simulink model "MARCH_v1_4"  (R2016a)
settings: Solver=FixedStepDiscrete  StartTime=0.0  StopTime=inf  FixedStep=0.001  RelTol=1e-3
InitFcn:
  | % Change dir to model location
  | cd(fileparts(which(bdroot)));
  | 
  | init_model
StartFcn:
  | cd(fileparts(which(bdroot)));
StopFcn:
  | cd(fileparts(which(bdroot)));
model workspace (MAT data in the model file):
  localValue = 1
  targetValue = 0
libraries: xpcethercatlib x61, slrtlib x7, dspnetwork x1, aerolibanimutils x1
(part 2 of 2)

== matlab function MARCH_v1_4/Controllers/Discrete Gait/Trajectory ==
  data: base input; q output; done output; trigger input; fullStep input; q input size=[1 6]; debugOut output; debugIn input
function [q,done,debugOut]= fcn(base,trigger,fullStep, q,debugIn)
%#codegen

persistent r splineCtrl i triggerPersistent torsoTrajectory trajectory hold fullWeightShift;

%% Initialize all variables
if(isempty(splineCtrl))
    splineCtrl = splineController();
end

if(isempty(fullWeightShift))
    fullWeightShift = 0;
end

if(isempty(fullStep))
    fullStep = 0;
end

if(isempty(r))
    % Get frequency of the model
    r = robotics();
    r.base = base;
    
end

if(isempty(hold))
    hold = 0;
end

if(isempty(i))
    i = 0;
end

if(isempty(triggerPersistent))
    triggerPersistent = trigger;
end


if(isempty(trajectory))
    trajectory = [0 0 0];
    torsoTrajectory = [0 0 0];
end

%% Logic
% Only run this for the beginning of the swing
r.torso_z = debugIn;

done = 0;

% Reset values if trigger is toggled.
if(triggerPersistent ~= trigger)
    r.base = base;
    i = 0;
    hold = 0;
    triggerPersistent = trigger;
end

% Hold exoskeleton in same position after a single step
if(hold)
    debugOut = r.torso_z;
    q = r.q;
    done = 1;
    return
end

if(~i)
    % Foot Trajectory
    splineCtrl.setStepHeight(0.5).setStepLength(0.3);
    if(~fullStep)
        trajectory = splineCtrl.method('circle').setVelocity(0.2).getHalfStep();
    else
        trajectory = splineCtrl.method('circle').setVelocity(0.2).getFullStep();
    end
    
    trajectory = r.transformSpline(trajectory);
    
    % Weight shift to base foot
    torso_delta = [0 0.1 0];
    
    if(r.base == 1)
        torso_delta(2) = abs(torso_delta(2));
    else
        torso_delta(2) = -abs(torso_delta(2));
    end
    
    if(~fullStep)
        torsoTrajectory = splineCtrl.getHalfWeightShift(torso_delta);
    else
        torsoTrajectory = splineCtrl.getFullWeightShift(torso_delta);
    end
    
    
    i = i+1;
end

r.point = [trajectory(1,i) trajectory(2,i) trajectory(3,i)];
r.step();
r.weightShift(torsoTrajectory(i,:));
r.inverseKinematics();

q = r.q;
debugOut = r.torso_z;

% Set final values as initial values for the next iteration
r.refresh();

% Reset iterator after we're done with the trajectory, otherwise we
% increment the counter and continue iterating as simulink continues
% sampling
if( i < (length(trajectory)))
    i = i+1;
else
    hold = 1;
end

end

== matlab function MARCH_v1_4/Controllers/Transition Controller/Torso Trajectory ==
  data: desired input; current input; z output
function z = fcn(desired, current)
%#codegen

persistent trajectory i desiredPersistent;

% Speed at which we home in SAMPLES
samples = 1000;

if (isempty(i))
    i = 0;
    
    % Hack to fix initial condition of delay during init phase
    current = desired;
end

if(isempty(desiredPersistent))
    desiredPersistent = desired;
end

if(isempty(trajectory))
    trajectory = linspace(current,desiredPersistent,samples);
end

if(desiredPersistent ~= desired)
    trajectory = linspace(current,desired,samples);
    desiredPersistent = desired;
    i = 0;
end

if(i < samples)
    i = i+1;
end

z = trajectory(i);

== matlab function MARCH_v1_4/Controllers/Transition Controller/Trajectory ==
  data: base input; q output; trigger input; q input size=[1 6]; debugOut output; debugIn input
function [q,debugOut]= fcn(base,trigger,q,debugIn)
%#codegen

persistent r splineCtrl i triggerPersistent trajectory fullStep hold;

%% Initialize all variables
if(isempty(splineCtrl))
    splineCtrl = splineController();
end


if(isempty(fullStep))
    fullStep = 0;
end

if(isempty(r))
    % Get frequency of the model
    r = robotics();
    r.base = base;
    
end

if(isempty(hold))
    hold = 0;
end

if(isempty(i))
    i = 0;
end

if(isempty(triggerPersistent))
    triggerPersistent = trigger;
end


if(isempty(trajectory))
    trajectory = [0 0];
end

%% Logic
% Only run this for the beginning of the swing
r.torso_z = debugIn;

% Reset values if trigger is toggled.
if(triggerPersistent ~= trigger)
    r.switchFoot(r.base);
    i = 0;
    hold = 0;
    triggerPersistent = trigger;
end

if(trigger == -1)
   fullStep = 0; 
end

% Hold exoskeleton in same position after a single step
if(hold)
    debugOut = r.torso_z;
    q = r.q;
    return
end

if(~i)
    
    % We set the method of whether we want an analytically generated spline
    % or a spline directly from the database.
    if(~fullStep)
        trajectory = splineCtrl.method('circle').getHalfStep();
        fullStep = 1;
    else
        trajectory = splineCtrl.method('circle').getFullStep();
    end
    
    % Transform the spline to the correct frame based on which foot is
    % swinging
    trajectory = r.transformSpline(trajectory);
    
    i = i+1;
end

r.point = [trajectory(1,i) trajectory(2,i) trajectory(3,i)];

r.stepPosture();
r.inverseKinematics();

q = r.q;
debugOut = r.torso_z;

% Set final values as initial values for the next iteration
r.refresh();

% Reset iterator after we're done with the trajectory, otherwise we
% increment the counter and continue iterating as simulink continues
% sampling
if( i < (length(trajectory)))
    i = i+1;
else
    hold = 1;
end

end

== matlab function MARCH_v1_4/Controllers/Point & Go/Trajectory ==
  data: base input; q output; trigger input; point input; q input size=[1 6]; debugOut output; debugIn input
function [q,debugOut]= fcn(base,trigger, point,q,debugIn)
%#codegen

persistent r splineCtrl i triggerPersistent trajectory fullStep hold pointPersistent;

%% Initialize all variables
if(isempty(splineCtrl))
    splineCtrl = splineController();
end


if(isempty(fullStep))
    fullStep = 0;
end

if(isempty(r))
    r = robotics();
    r.base = base;
    
end

if(isempty(hold))
    hold = 0;
end

if(isempty(i))
    i = 0;
end

if(isempty(triggerPersistent))
    triggerPersistent = trigger;
end

if(isempty(pointPersistent))
    pointPersistent = point;
end

if(isempty(trajectory))
    trajectory = [0 0];
end

%% Logic

% Reset values if trigger is toggled.
if(triggerPersistent ~= trigger)
    r.base = base;
    i = 0;
    hold = 0;
    triggerPersistent = trigger;
end


% Hold exoskeleton in same position after a single step
if(hold)
    debugOut = r.torso_z;
    q = r.q;
    return
end

if(~i)
    
    % We set the method of whether we want an analytically generated spline
    % or a spline directly from the database.
    % Options: 'circle' and 'stairs'
    splineCtrl.setStepHeight(0.3);
    trajectory = splineCtrl.method('circle').getStepFromPoint(point);
    
    
    
    % Transform the spline to the correct frame based on which foot is
    % swinging
    trajectory = r.transformSpline(trajectory);
    
    i = i+1;
end

r.point = [trajectory(1,i) trajectory(2,i) trajectory(3,i)];

r.stepPosture();
r.inverseKinematics();

q = r.q;
debugOut = r.torso_z;

% Set final values as initial values for the next iteration
r.refresh();

% Reset iterator after we're done with the trajectory, otherwise we
% increment the counter and continue iterating as simulink continues
% sampling
if( i < (length(trajectory)))
    i = i+1;
else
    hold = 1;
end

end

== matlab function MARCH_v1_4/EtherCAT Joint Setpoints/exoskeleton/MATLAB Function ==
  data: jointAngle input; encVal output; par parameter
function encVal = convertToEncoderValues(jointAngle, par)
encVal = zeros(6,1);

for i = 1:6
    encVal(i) = rad2enc(jointAngle(i), i, par);
end

== matlab function MARCH_v1_4/Controllers/Stand/Trajectory ==
  data: q output; trigger input; q_i input size=[1 6]; debugIn input
function q = fcn(trigger,q_i,debugIn)
%#codegen

persistent r splineCtrl i q_t;

%% Initialize all variables
if(isempty(splineCtrl))
    splineCtrl = splineController();
end

if(isempty(r))
    % Get frequency of the model
    r = robotics();
    
end

if(isempty(q_t))
   q_t = [0 0 0 0 0 0];
end

if(isempty(i))
    i = 0;
end


%% Logic

if(~i)
    q_f = [0 0 0 0 0 0];
    splineCtrl.samples = 4000;
    q_t = splineCtrl.getStandupJointTrajectory(q_i,q_f);
    
    i = i+1;
end

q = q_t(i,:);

if( i < length(q_t))
    i = i+1;
end

end

== matlab function MARCH_v1_4/State Machine/Trigger Function ==
  data: base output; right input; trigger output; left input
function [base,trigger] = fcn(right,left)
%#codegen

persistent triggerPersistent hold;

if(isempty(triggerPersistent))
    triggerPersistent = 0;
end

if(isempty(hold))
    hold = 0;
end

trigger = triggerPersistent;


% If both left and right are equal don't do anything
if(left == right)
    trigger = triggerPersistent;
    hold = 0;
end

% If right and left differ, toggle trigger
if(left ~= right && ~hold)
    trigger = 1 - triggerPersistent;
    hold = 1;
end

if(left)
    base = 1;
else
    base = 3;
end


triggerPersistent = trigger;

== matlab function MARCH_v1_4/Controllers/Stairs/Torso Trajectory ==
  data: desired input; torsoTrajectory output size=[1 3]
function torsoTrajectory = fcn(desired)
%#codegen

persistent trajectory i desiredPersistent;

% Speed at which we home in SAMPLES
samples = 1000;

if (isempty(i))
    i = 0;
end

if(isempty(desiredPersistent))
    desiredPersistent = desired;
end

if(isempty(trajectory))   
    desiredPersistent = desired;
    
    trajectory = [linspace(0,desiredPersistent(1),samples)
        linspace(0,desiredPersistent(2),samples)
        linspace(0,desiredPersistent(3),samples) ]';
end

if(~isequal(desiredPersistent,desired))
    trajectory = [linspace(0,desired(1),samples)
        linspace(0,desired(2),samples)
        linspace(0,desired(3),samples) ]';
    
    desiredPersistent = desired;
    i = 0;
end

if(i < samples)
    i = i+1;
end

torsoTrajectory = trajectory(i,:);

== matlab function MARCH_v1_4/Controllers/Stairs/Trajectory ==
  data: base input; q output; trigger_t input; q input size=[1 6]; torso_delta input size=[1 3]
function q  = fcn(base,trigger_t,q,torso_delta)
%#codegen

persistent r s i j trigger trajectory torsoTrajectory seq;

%% Initialize all variables
if(isempty(s))
    s = splineController();
end

if(isempty(r))
    % Get frequency of the model
    r = robotics();
    r.base = base;
    
end

if(isempty(seq))
    seq = 1;
end

if(isempty(i) || isempty(j))
    i = 0;
    j = 0;
end

if(isempty(trigger))
    trigger = trigger_t;
end

if(isempty(torsoTrajectory))
    torsoTrajectory = [0 0 0];
end

if(isempty(trajectory))
    trajectory = [0 0 0];
end

%% Weight shifting sequence
% This sequence will weight shift to the base leg. The entire sequence is
% wrapped inside an if statement to prevent this from executing after it
% has been completed. It is either this or a separate function block which
% would be a disaster because the classes are separate instances.
if(seq == 1)
    if (~i)
        r.setTorsoHeight(0.95);
        r.refresh(); % make sure initial position of torso has same heighit as set above
        % Override sample speed
        s.samples = 1000;
        
        % Weight shift to base foot
        if(base == 1)
            torso_delta(2) = -abs(torso_delta(2));
        else
            torso_delta(2) = abs(torso_delta(2));
        end
        
        torsoTrajectory = s.getHalfWeightShift(torso_delta);
        i = i+1;
    end
    
    % Playback trajectory and return preventing doing the rest
    if(i < length(torsoTrajectory))
        r.reset();
        r.weightShift(torsoTrajectory(i,:));
        r.inverseKinematics();
        q = r.q;
        
        i = i+1;
        return
    else
        q = r.q;
        
        % Init and enable step sequence
        r.refresh();
        j = 0;
        % Disable weight shifting
        seq = 2;
    end
end

%% Step Sequence
% This sequence will step onto the stair
if(seq == 2)
    if(~j)
        s.setStepHeight(0.2).setStepLength(0.5);
        
        trajectory = s.method('circle').setVelocity(0.21).getHalfStep();
        trajectory = r.transformSpline(trajectory);
        if(r.base == 1)
            torso_delta(2) = -abs(torso_delta(2));
        else
            torso_delta(2) = abs(torso_delta(2));
        end
        % Shift the weight back to the middle during the step
        torsoTrajectory = s.getWeightShift(torso_delta, [0 0 0]);
        
        j = j+1;
    end
    
    r.point = [trajectory(1,j) trajectory(2,j) trajectory(3,j)];
    r.step();

    % Weight shift the torso back to the middle
    r.weightShift(torsoTrajectory(j,:));
    r.inverseKinematics();
    
    q = r.q;
    
    % THIS SHOULD NOT BE HERE BUT IT WON'T WORK OTHERWISE :(
    r.refresh();
    
    if(j < length(trajectory))
        j = j+1;
    else
        j = 0;
        q = r.q;
        r.switchFoot(r.base);
    end
    
end
end

== matlab function MARCH_v1_4/Controllers/0-Torque/RHAA/Sample and Hold ==
  data: offset input; reference output
function reference = fcn(offset)
%#codegen

persistent offsetPersistent;

if(isempty(offsetPersistent))
    offsetPersistent = uint32(0);
end

if(offset > 0)
    
    offsetPersistent = offset;
    
end

reference = offsetPersistent;
